simulink model "Modulador_torque"  (R2020b)
settings: Solver=ode23s  StartTime=0.0  StopTime=30  RelTol=1e-3
undefined symbols (not defined in the file): alfa_cu, Beq, Cts, Jeq, K_i_o, K_omega_o, K_tita_o, Kd, Ki, Kp, lambda_m, Ld, Lls, Lq, Pp, r, R0, R_Ref, Rd, Rq, Rts_amb, sigbuilder_block, TREF
libraries: simulink x2
settings Model: Creator=agustin  LastModifiedBy=emaag

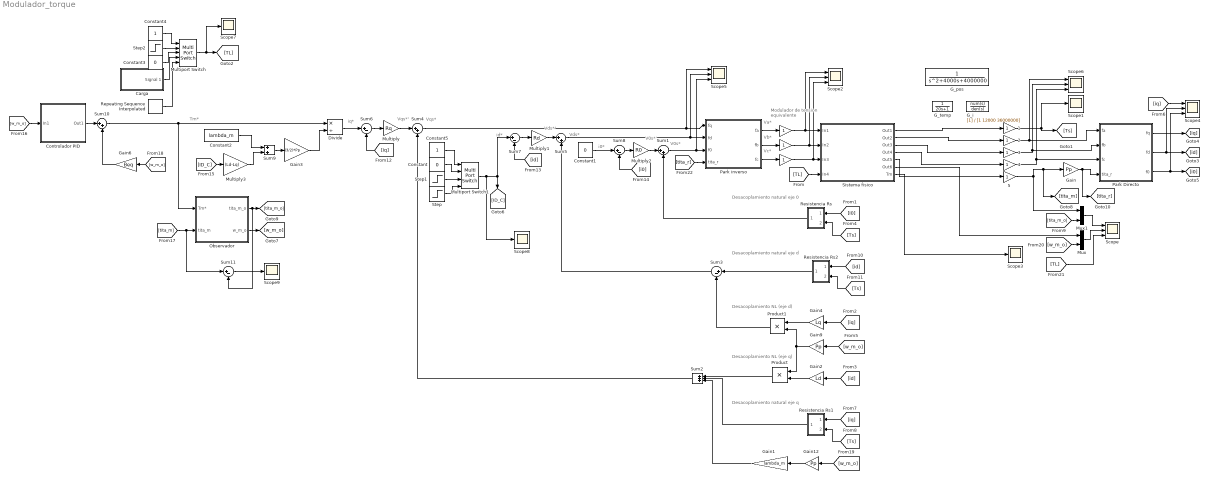
== system Modulador_torque ==
  note: Tm*
  note: V0s*'
  note: Vds*'
  note: Vqs*'
  note: i0*
  note: id*
  note: iq*
  note: V0s*
  note: Vds*
  note: Vb*
  note: Vc*
  note: Va*
  note: Desacoplamiento NL (eje q)
  note: Desacoplamiento NL (eje d)
  note: Vqs*
  note: Modulador de tension
      | equivalente
  note: Desacoplamiento natural eje 0
  note: Desacoplamiento natural eje q
  note: Desacoplamiento natural eje d
   {,,,1..5} (8 alike) : Gain
  Carga : Subsystem  Tag=STV Subsys  LoadFcn=sigbuilder_block('load');  StartFcn=sigbuilder_block('start');  StopFcn=sigbuilder_block('stop');  ClipboardFcn=sigbuilder_block('clipboard');  mask(Sigbuilder block){tuvar=[0:10]}
      mask help: Simulink:masks:SigbuilderBlock_MD
      mask init:
      | if ~strcmp(get_param(bdroot(gcbh),'SimulationStatus'),'stopped') tuvar = sigbuilder_block('maskInit'); end
      settings: CopyFcn=sigbuilder_block('copy');  DeleteFcn=sigbuilder_block('delete');  ModelCloseFcn=sigbuilder_block('modelClose');  PreSaveFcn=sigbuilder_block('preSave');  PauseFcn=sigbuilder_block('pause');  ContinueFcn=sigbuilder_block('continue');  NameChangeFcn=sigbuilder_block('namechange');  OpenFcn=sigbuilder_block('open',[6 30 1012.5 447.75 ]);  CloseFcn=sigbuilder_block('close');
      mask Display: plot(0, 0, 100, 100,[2, 2, 32, 32, 2], [68, 8, 8, 68, 68],[32, 2], [38, 38], [32, 19, 2],[53, 60, 44], [32, 17, 17, 2],[16, 16, 31, 31]);txt = getActiveGroup(gcbh);text(2, 100, txt,'verticalAlignment', 'top');
  Constant : Constant  Value=0
  Constant1 : Constant  Value=0
  Constant2 : Constant  Value=lambda_m
  Constant3 : Constant  Value=0
  Constant4 : Constant
  Constant5 : Constant
  Controlador PID : Subsystem
  Divide : Product  Inputs=*/
  G_i : TransferFcn  Denominator=[1 12000 36000000]
  G_pos : TransferFcn  Denominator=[1 4000 4000000]
  G_temp : TransferFcn  Denominator=[20 1]
  Gain : Gain  Gain=Pp
  Gain1 : Gain  Gain=lambda_m
  Gain12 : Gain  Gain=Pp
  Gain2 : Gain  Gain=Ld
  Gain3 : Gain  Gain=(3/2)*Pp
  Gain4 : Gain  Gain=Lq
  Gain6 : Gain  Gain=Beq
  Gain9 : Gain  Gain=Pp
  Multiply : Gain  Gain=Rq
  Multiply1 : Gain  Gain=Rd
  Multiply2 : Gain  Gain=R0
  Multiply3 : Gain  Gain=(Ld-Lq)
  Multiport Switch : MultiPortSwitch  Inputs=4
  Multiport Switch1 : MultiPortSwitch
  Mux : Mux  Inputs=2
  Mux1 : Mux  Inputs=2
  Observador : Subsystem
  Park Directo : MATLAB Function  TreatAsAtomicUnit=on
  Park inverso : MATLAB Function  TreatAsAtomicUnit=on
  Product : Product
  Product1 : Product
  Repeating Sequence Interpolated : simulink/Sources/Repeating Sequence Interpolated  OutValues="[0 0 6.28 6.28 -6.28 -6.28 0  0].'"  TimeValues="[0 .3 .30000001 .5 .5000001 .9 .9000001  10].'"  LookUpMeth=Interpolation-Use End Values  tsamp=0.01  OutMin=[]  OutMax=[]  OutDataTypeStr=double  OutputDataTypeScalingMode=double  OutDataType=fixdt(0,8)  OutScaling=2^-10
  Resistencia Rs : Subsystem
  Resistencia Rs1 : Subsystem
  Resistencia Rs2 : Subsystem
  Scope{,2,4..6} (5 alike) : Scope  NumInputPorts=3
  Scope{1,3,7..9} (5 alike) : Scope
  Sistema fisico : Subsystem
  Step : Step  Time=0.5  After=-1.9596  SampleTime=0
  Step1 : Step  Time=0.5  After=1.9596  SampleTime=0
  Step2 : Step  Time=3  After=6.28  SampleTime=0
  Sum{1,4..5,10} (4 alike) : Sum  Inputs=|++
  Sum{3,6..8,11} (5 alike) : Sum  Inputs=|+-
  Sum2 : Sum  Inputs=+++
  Sum9 : Sum
  wires:
  Sum5/1 -> Park inverso/2(fd), Scope5/2
  " 1"/1 -> [Ts], Scope1/1
  Gain4/1 -> Product1/1
  Park inverso/3(fc) -> " "/1
  Park inverso/1(fa) -> " "/1
  Sistema fisico/1(Out1) -> " 1"/1
  Park Directo/3(f0) -> Scope4/3, [i0]
  Sum1/1 -> Park inverso/3(f0), Scope5/3
  Gain/1 -> [tita_r], Park Directo/4(tita_r)
  [iq] -> Scope4/1
  Sistema fisico/4(Out4) -> " 4"/1
  [id] -> Gain2/1
  Sistema fisico/6(Out6) -> Mux/1
  " "/1 -> Scope2/2, Sistema fisico/2(In2)
  Sum4/1 -> Scope5/1, Park inverso/1(fq)
  [iq] -> Gain4/1
  " 3"/1 -> Scope6/2, Park Directo/2(fb)
  " "/1 -> Scope2/3, Sistema fisico/3(In3)
  [TL] -> Sistema fisico/4(In4)
  Sistema fisico/3(Out3) -> " 3"/1
  Park inverso/2(fb) -> " "/1
  " "/1 -> Sistema fisico/1(In1), Scope2/1
  Park Directo/2(fd) -> Scope4/2, [id]
  Sistema fisico/5(Out5) -> " 5"/1
  Sistema fisico/7(Tm) -> Scope3/1
  Gain2/1 -> Product/2
  " 4"/1 -> Scope6/3, Park Directo/3(fc)
  Sistema fisico/2(Out2) -> " 2"/1
  Park Directo/1(fq) -> [iq]
  " 2"/1 -> Scope6/1, Park Directo/1(fa)
  [i0] -> Resistencia Rs/1(In1)
  Resistencia Rs/1(In*Rs) -> Sum1/2
  [Ts] -> Resistencia Rs/2(Ts)
  [iq] -> Resistencia Rs1/1(In1)
  Resistencia Rs1/1(In*Rs) -> Sum2/2
  [Ts] -> Resistencia Rs1/2(Ts)
  Gain12/1 -> Gain1/1
  Sum2/1 -> Sum4/2
  [Ts] -> Resistencia Rs2/2(Ts)
  [id] -> Resistencia Rs2/1(In1)
  Sum3/1 -> Sum5/2
  Resistencia Rs2/1(In*Rs) -> Sum3/1
  Sum6/1 -> Multiply/1
  [iq] -> Sum6/2
  [id] -> Sum7/2
  [i0] -> Sum8/2
  Multiply/1 -> Sum4/1
  Multiply1/1 -> Sum5/1
  Sum7/1 -> Multiply1/1
  Sum8/1 -> Multiply2/1
  Multiply2/1 -> Sum1/1
  Product1/1 -> Sum3/2
  Product/1 -> Sum2/1
  Gain1/1 -> Sum2/3
  Step1/1 -> Multiport Switch1/3
  Constant/1 -> Multiport Switch1/2
  Step/1 -> Multiport Switch1/4
  Multiport Switch1/1 -> Scope8/1, [ID_C], Sum7/1
  Constant1/1 -> Sum8/1
  [ID_C] -> Multiply3/1
  Multiply3/1 -> Sum9/2
  Constant2/1 -> Sum9/1
  Sum9/1 -> Gain3/1
  Gain3/1 -> Divide/2
  Divide/1 -> Sum6/1
  Gain6/1 -> Sum10/2
  Constant3/1 -> Multiport Switch/3
  Carga/1(Signal 1) -> Multiport Switch/4
  Multiport Switch/1 -> Scope7/1, [TL]
  [w_m_o] -> Controlador PID/1(In1)
  " 5"/1 -> [tita_m], Gain/1, Mux1/1
  Sum10/1 -> Divide/1, Observador/1(Tm*)
  [w_m_o] -> Gain6/1
  [w_m_o] -> Gain9/1
  Gain9/1 -> Product1/2, Product/1
  [w_m_o] -> Gain12/1
  [tita_m_o] -> Mux1/2
  [w_m_o] -> Mux/2
  Mux1/1 -> Scope/1
  Mux/1 -> Scope/2
  [TL] -> Scope/3
  Step2/1 -> Multiport Switch/2
  Controlador PID/1(Out1) -> Sum10/1
  Constant4/1 -> Multiport Switch/1
  Constant5/1 -> Multiport Switch1/1
  [tita_m] -> Sum11/1, Observador/2(tita_m)
  Observador/1(tita_m_o) -> Sum11/2, [tita_m_o]
  Observador/2(w_m_o) -> [w_m_o]
  [tita_r] -> Park inverso/4(tita_r)
  Repeating Sequence Interpolated/1 -> Multiport Switch/5
  Sum11/1 -> Scope9/1

== system Modulador_torque/Carga ==
  Demux : Demux  Tag=STV Demux  Outputs=1
      settings: DisplayOption=none
  FromWs : FromWorkspace  Tag=STV FromWs  VariableName=tuvar
      SigBuilderData=|
      | common.afterFinalStr = 'Extrapolate'
      | common.sampleTime = 0
      | dataSet.timeRange = [0 10]
      | dataSet.name = 'Group 1'
      | sbobj.Groups.Name = 'Group 1'
      | sbobj.Groups.Signals.Name = 'Signal 1'
      | sbobj.Groups.Signals.XData = [0 0.3 0.3 0.5 0.5 0.9 0.9 10]
      | sbobj.Groups.Signals.YData = [0 0 6.28 6.28 -6.28 -6.28 0 0]
  Signal 1 : Outport  Tag=STV Outport  VectorParamsAs1DForOutWhenUnconnected=off
  wires:
  Demux/1 -> Signal 1/1
  FromWs/1 -> Demux/1

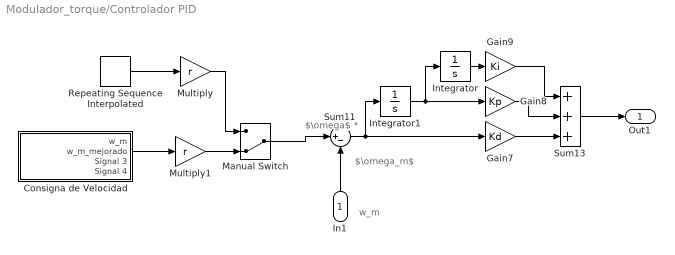
== system Modulador_torque/Controlador PID ==
  note: w_m
  note: $\omega_m$
  note: $\omega$ *
  In1 : Inport
  Consigna de Velocidad : Subsystem  Tag=STV Subsys  LoadFcn=sigbuilder_block('load');  StartFcn=sigbuilder_block('start');  StopFcn=sigbuilder_block('stop');  ClipboardFcn=sigbuilder_block('clipboard');  mask(Sigbuilder block){tuvar=[0:10]}
      mask help: Simulink:masks:SigbuilderBlock_MD
      mask init:
      | if ~strcmp(get_param(bdroot(gcbh),'SimulationStatus'),'stopped') tuvar = sigbuilder_block('maskInit'); end
      settings: CopyFcn=sigbuilder_block('copy');  DeleteFcn=sigbuilder_block('delete');  ModelCloseFcn=sigbuilder_block('modelClose');  PreSaveFcn=sigbuilder_block('preSave');  PauseFcn=sigbuilder_block('pause');  ContinueFcn=sigbuilder_block('continue');  NameChangeFcn=sigbuilder_block('namechange');  OpenFcn=sigbuilder_block('open',[6 30 1012.5 447.75 ]);  CloseFcn=sigbuilder_block('close');
      mask Display: plot(0, 0, 100, 100,[2, 2, 32, 32, 2], [68, 8, 8, 68, 68],[32, 2], [38, 38], [32, 19, 2],[53, 60, 44], [32, 17, 17, 2],[16, 16, 31, 31]);txt = getActiveGroup(gcbh);text(2, 100, txt,'verticalAlignment', 'top');
  Gain7 : Gain  Gain=Kd
  Gain8 : Gain  Gain=Kp
  Gain9 : Gain  Gain=Ki
  Integrator : Integrator
  Integrator1 : Integrator
  Manual Switch : ManualSwitch  CurrentSetting=0
  Multiply : Gain  Gain=r
  Multiply1 : Gain  Gain=r
  Repeating Sequence Interpolated : simulink/Sources/Repeating Sequence Interpolated  OutValues="[0 0 1.2566 1.2566 0  0 -1.2566 -1.2566 0 0].'"  TimeValues=[0 4.7 5 10 10.3 14.7 15 20 20.3 25].'  LookUpMeth=Interpolation-Use End Values  tsamp=0.01  OutMin=[]  OutMax=[]  OutDataTypeStr=double  OutputDataTypeScalingMode=double  OutDataType=fixdt(0,8)  OutScaling=2^-10
  Sum11 : Sum  Inputs=|+-
  Sum13 : Sum  Inputs=+++
  Out1 : Outport
  wires:
  Gain9/1 -> Sum13/1
  Sum11/1 -> Integrator1/1, Gain7/1
  Sum13/1 -> Out1/1
  Integrator1/1 -> Integrator/1, Gain8/1
  Gain8/1 -> Sum13/2
  Integrator/1 -> Gain9/1
  Gain7/1 -> Sum13/3
  In1/1 -> Sum11/2
  Manual Switch/1 -> Sum11/1
  Repeating Sequence Interpolated/1 -> Multiply/1
  Multiply/1 -> Manual Switch/1
  Consigna de Velocidad/2(w_m_mejorado) -> Multiply1/1
  Multiply1/1 -> Manual Switch/2

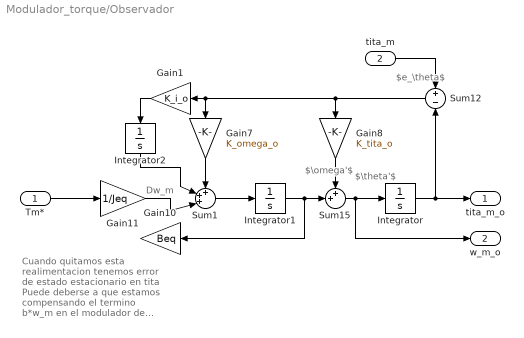
== system Modulador_torque/Observador ==
  note: $\omega'$
  note: $\theta'$
  note: $e_\theta$
  note: Cuando quitamos esta realimentacion tenemos error de estado estacionario en tita
      | Puede deberse a que estamos compensando el termino b*w_m en el modulador de torque
  note: Dw_m
  Tm* : Inport
  tita_m : Inport  Port=2
  Gain1 : Gain  Gain=K_i_o
  Gain10 : Gain  Gain=Beq
  Gain11 : Gain  Gain=1/Jeq
  Gain7 : Gain  Gain=K_omega_o
  Gain8 : Gain  Gain=K_tita_o
  Integrator : Integrator
  Integrator1 : Integrator
  Integrator2 : Integrator
  Sum1 : Sum  Inputs=+++|
  Sum12 : Sum  Inputs=+-
  Sum15 : Sum  Inputs=++|
  tita_m_o : Outport
  w_m_o : Outport  Port=2
  wires:
  Gain8/1 -> Sum15/1
  Integrator/1 -> tita_m_o/1, Sum12/2
  Sum1/1 -> Integrator1/1
  Integrator1/1 -> Sum15/2, Gain10/1
  Sum12/1 -> Gain1/1, Gain7/1, Gain8/1
  Sum15/1 -> w_m_o/1, Integrator/1
  tita_m/1 -> Sum12/1
  Tm*/1 -> Gain11/1
  Gain1/1 -> Integrator2/1
  Gain7/1 -> Sum1/1
  Integrator2/1 -> Sum1/2
  Gain11/1 -> Sum1/3

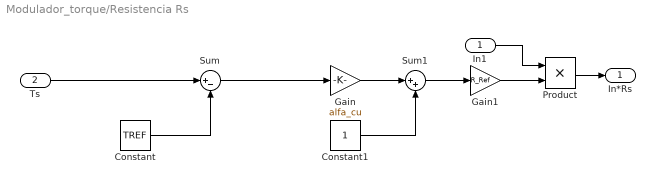
== system Modulador_torque/Resistencia Rs ==
  In1 : Inport
  Ts : Inport  Port=2
  Constant : Constant  Value=TREF
  Constant1 : Constant
  Gain : Gain  Gain=alfa_cu
  Gain1 : Gain  Gain=R_Ref
  Product : Product
  Sum : Sum  Inputs=|+-
  Sum1 : Sum  Inputs=|++
  In*Rs : Outport
  wires:
  Constant/1 -> Sum/2
  Gain/1 -> Sum1/1
  Gain1/1 -> Product/2
  Sum1/1 -> Gain1/1
  Sum/1 -> Gain/1
  Ts/1 -> Sum/1
  Constant1/1 -> Sum1/2
  In1/1 -> Product/1
  Product/1 -> In*Rs/1

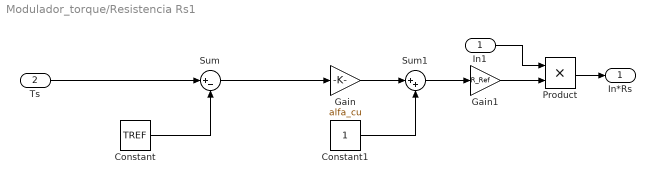
== system Modulador_torque/Resistencia Rs1 ==
  In1 : Inport
  Ts : Inport  Port=2
  Constant : Constant  Value=TREF
  Constant1 : Constant
  Gain : Gain  Gain=alfa_cu
  Gain1 : Gain  Gain=R_Ref
  Product : Product
  Sum : Sum  Inputs=|+-
  Sum1 : Sum  Inputs=|++
  In*Rs : Outport
  wires:
  Constant/1 -> Sum/2
  Gain/1 -> Sum1/1
  Gain1/1 -> Product/2
  Sum1/1 -> Gain1/1
  Sum/1 -> Gain/1
  Ts/1 -> Sum/1
  Constant1/1 -> Sum1/2
  In1/1 -> Product/1
  Product/1 -> In*Rs/1

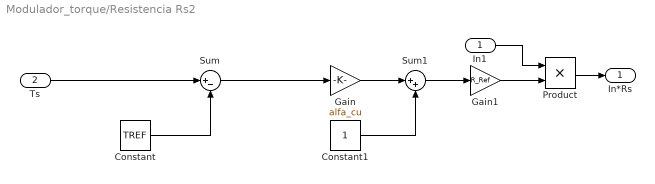
== system Modulador_torque/Resistencia Rs2 ==
  In1 : Inport
  Ts : Inport  Port=2
  Constant : Constant  Value=TREF
  Constant1 : Constant
  Gain : Gain  Gain=alfa_cu
  Gain1 : Gain  Gain=R_Ref
  Product : Product
  Sum : Sum  Inputs=|+-
  Sum1 : Sum  Inputs=|++
  In*Rs : Outport
  wires:
  Constant/1 -> Sum/2
  Gain/1 -> Sum1/1
  Gain1/1 -> Product/2
  Sum1/1 -> Gain1/1
  Sum/1 -> Gain/1
  Ts/1 -> Sum/1
  Constant1/1 -> Sum1/2
  In1/1 -> Product/1
  Product/1 -> In*Rs/1

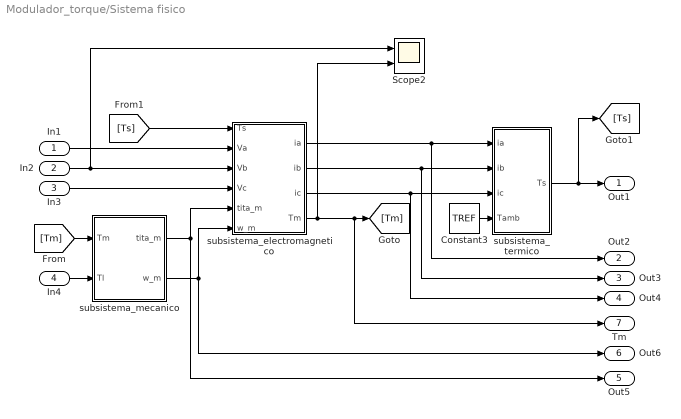
== system Modulador_torque/Sistema fisico ==
  In1 : Inport
  In2 : Inport  Port=2
  In3 : Inport  Port=3
  In4 : Inport  Port=4
  Constant3 : Constant  Value=TREF
  Scope2 : Scope  NumInputPorts=2
  "subsistema_electromagnetico " : Subsystem
  "subsistema_mecanico " : Subsystem
  subsistema_termico : Subsystem
  Out1 : Outport  VectorParamsAs1DForOutWhenUnconnected=off
  Out2 : Outport  Port=2  VectorParamsAs1DForOutWhenUnconnected=off
  Out3 : Outport  Port=3  VectorParamsAs1DForOutWhenUnconnected=off
  Out4 : Outport  Port=4  VectorParamsAs1DForOutWhenUnconnected=off
  Out5 : Outport  Port=5  VectorParamsAs1DForOutWhenUnconnected=off
  Out6 : Outport  Port=6  VectorParamsAs1DForOutWhenUnconnected=off
  Tm : Outport  Port=7  VectorParamsAs1DForOutWhenUnconnected=off
  wires:
  "subsistema_mecanico "/2(w_m) -> Out6/1, "subsistema_electromagnetico "/6(w_m)
  "subsistema_electromagnetico "/3(ic) -> Out4/1, subsistema_termico/3("ic ")
  In2/1 -> Scope2/1, "subsistema_electromagnetico "/3(Vb)
  [Tm] -> "subsistema_mecanico "/1(Tm)
  In4/1 -> "subsistema_mecanico "/2(Tl)
  "subsistema_electromagnetico "/1(ia) -> Out2/1, subsistema_termico/1(ia)
  "subsistema_electromagnetico "/4(Tm) -> Scope2/2, Tm/1, [Tm]
  In1/1 -> "subsistema_electromagnetico "/2(Va)
  Constant3/1 -> subsistema_termico/4(Tamb)
  "subsistema_electromagnetico "/2(ib) -> Out3/1, subsistema_termico/2(ib)
  In3/1 -> "subsistema_electromagnetico "/4(Vc)
  "subsistema_mecanico "/1("tita_m ") -> Out5/1, "subsistema_electromagnetico "/5(tita_m)
  subsistema_termico/1(Ts) -> [Ts], Out1/1
  [Ts] -> "subsistema_electromagnetico "/1(Ts)

== system Modulador_torque/Controlador PID/Consigna de Velocidad ==
  Demux : Demux  Tag=STV Demux
      settings: DisplayOption=none
  FromWs : FromWorkspace  Tag=STV FromWs  VariableName=tuvar
      SigBuilderData=|
      | common.afterFinalStr = 'Extrapolate'
      | common.sampleTime = 0
      | dataSet.timeRange = [0 25]
      | dataSet.name = 'Group 1'
      | sbobj.Groups.Name = 'Group 1'
      | sbobj.Groups.Signals(1).Name = 'w_m'
      | sbobj.Groups.Signals(1).XData = [0 5 5 10 10 15 15 20 20 25]
      | sbobj.Groups.Signals(1).YData = [0 0 1.2566 1.25660004683 0 0 -1.2566 -1.2566 0 0]
      | sbobj.Groups.Signals(2).Name = 'w_m_mejorado'
      | sbobj.Groups.Signals(2).XData = [0 4.7 5 10 10.3 14.7 15 20 20.3 25]
      | sbobj.Groups.Signals(2).YData = [0 0 1.25660004683 1.25660004683 0 0 -1.25660004683 -1.25660004683 0 0]
      | sbobj.Groups.Signals(3).Name = 'Signal 3'
      | sbobj.Groups.Signals(3).XData = [0 3.28 6 6 9 9 11.94 25]
      | sbobj.Groups.Signals(3).YData = [0 0 0 1 1 0 0 0]
      | sbobj.Groups.Signals(4).Name = 'Signal 4'
      | sbobj.Groups.Signals(4).XData = [0 6.8 6.8 10.2 10.2 25]
      | sbobj.Groups.Signals(4).YData = [0 0 1 1 0 0]
      | sbobj.Groups.TimeRange = [0 25]
  w_m : Outport  Tag=STV Outport  VectorParamsAs1DForOutWhenUnconnected=off
  w_m_mejorado : Outport  Tag=STV Outport  Port=2
  Signal 3 : Outport  Tag=STV Outport  Port=3
  Signal 4 : Outport  Tag=STV Outport  Port=4
  wires:
  Demux/1 -> w_m/1
  FromWs/1 -> Demux/1
  Demux/2 -> w_m_mejorado/1
  Demux/3 -> Signal 3/1
  Demux/4 -> Signal 4/1

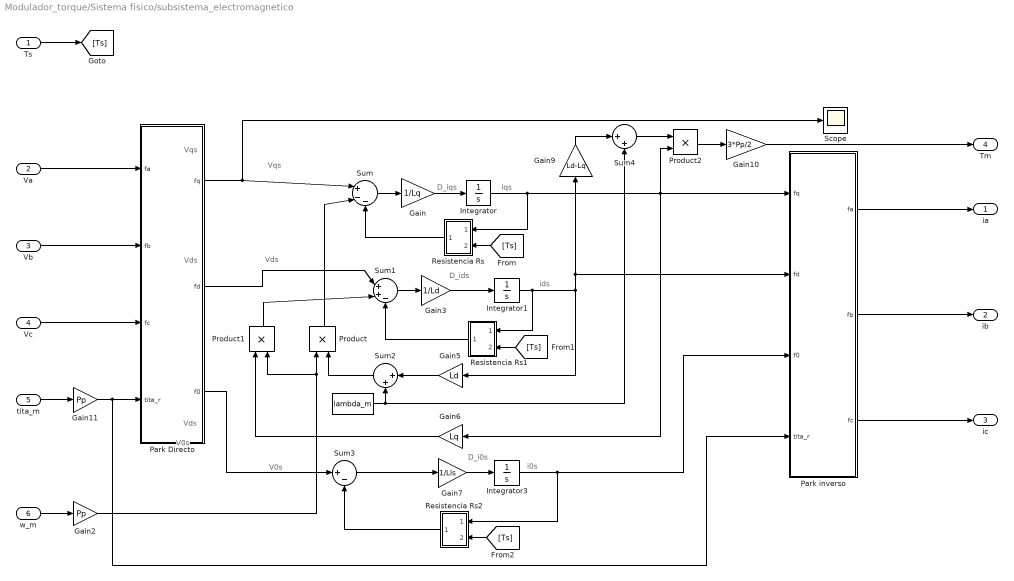
== system Modulador_torque/Sistema fisico/subsistema_electromagnetico  ==
  note: V0s
  note: Vds
  note: Vqs
  note: Vds
  note: Vqs
  note: V0s
  note: Vds
  note: i0s
  note: D_i0s
  note: D_ids
  note: ids
  note: iqs
  note: D_iqs
  Ts : Inport
  Va : Inport  Port=2
  Vb : Inport  Port=3
  Vc : Inport  Port=4
  tita_m : Inport  Port=5
  w_m : Inport  Port=6
  " " : Constant  Value=lambda_m
  Gain : Gain  Gain=1/Lq
  Gain10 : Gain  Gain=3*Pp/2
  Gain11 : Gain  Gain=Pp
  Gain2 : Gain  Gain=Pp
  Gain3 : Gain  Gain=1/Ld
  Gain5 : Gain  Gain=Ld
  Gain6 : Gain  Gain=Lq
  Gain7 : Gain  Gain=1/Lls
  Gain9 : Gain  Gain=Ld-Lq
  Integrator : Integrator
  Integrator1 : Integrator
  Integrator3 : Integrator
  Park Directo : MATLAB Function  TreatAsAtomicUnit=on
  Park inverso : MATLAB Function  TreatAsAtomicUnit=on
  Product : Product
  Product1 : Product
  Product2 : Product
  Resistencia Rs : Subsystem
  Resistencia Rs1 : Subsystem
  Resistencia Rs2 : Subsystem
  Scope : Scope
  Sum : Sum  Inputs=|+--
  Sum1 : Sum  Inputs=|++-
  Sum2 : Sum  Inputs=|++
  Sum3 : Sum  Inputs=|+-
  Sum4 : Sum  Inputs=|++
  ia : Outport  VectorParamsAs1DForOutWhenUnconnected=off
  ib : Outport  Port=2  VectorParamsAs1DForOutWhenUnconnected=off
  ic : Outport  Port=3  VectorParamsAs1DForOutWhenUnconnected=off
  Tm : Outport  Port=4  VectorParamsAs1DForOutWhenUnconnected=off
  wires:
  Product/1 -> Sum/2
  w_m/1 -> Gain2/1
  Product1/1 -> Sum1/2
  Gain2/1 -> Product1/2, Product/1
  Park Directo/3(f0) -> Sum3/1
  Integrator/1 -> Resistencia Rs/1(In1), Product2/2, Park inverso/1(fq), Gain6/1
  Sum2/1 -> Product/2
  Sum3/1 -> Gain7/1
  Park Directo/1(fq) -> Scope/1, Sum/1
  Sum/1 -> Gain/1
  Gain3/1 -> Integrator1/1
  Park Directo/2(fd) -> Sum1/1
  Sum1/1 -> Gain3/1
  Gain5/1 -> Sum2/1
  Gain/1 -> Integrator/1
  Gain6/1 -> Product1/1
  Resistencia Rs/1(In*Rs) -> Sum/3
  " "/1 -> Sum4/2, Sum2/2
  Gain7/1 -> Integrator3/1
  Gain9/1 -> Sum4/1
  Sum4/1 -> Product2/1
  Product2/1 -> Gain10/1
  Gain10/1 -> Tm/1
  Vb/1 -> Park Directo/2(fb)
  Va/1 -> Park Directo/1(fa)
  Vc/1 -> Park Directo/3(fc)
  tita_m/1 -> Gain11/1
  Gain11/1 -> Park inverso/4(tita_r), Park Directo/4(tita_r)
  Park inverso/1(fa) -> ia/1
  Park inverso/2(fb) -> ib/1
  Park inverso/3(fc) -> ic/1
  Ts/1 -> [Ts]
  [Ts] -> Resistencia Rs/2(Ts)
  Resistencia Rs1/1(In*Rs) -> Sum1/3
  Integrator1/1 -> Gain9/1, Park inverso/2(fd), Gain5/1, Resistencia Rs1/1(In1)
  [Ts] -> Resistencia Rs1/2(Ts)
  Resistencia Rs2/1(In*Rs) -> Sum3/2
  Integrator3/1 -> Resistencia Rs2/1(In1), Park inverso/3(f0)
  [Ts] -> Resistencia Rs2/2(Ts)

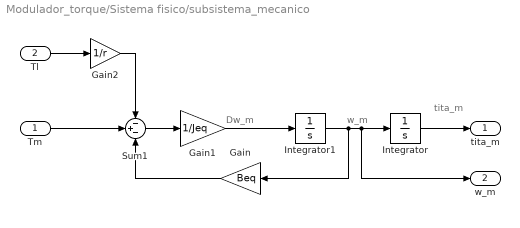
== system Modulador_torque/Sistema fisico/subsistema_mecanico  ==
  note: Dw_m
  note: w_m
  note: tita_m
  Tm : Inport
  Tl : Inport  Port=2
  Gain : Gain  Gain=Beq
  Gain1 : Gain  Gain=1/Jeq
  Gain2 : Gain  Gain=1/r
  Integrator : Integrator
  Integrator1 : Integrator
  Sum1 : Sum  Inputs=-+-
  "tita_m " : Outport  VectorParamsAs1DForOutWhenUnconnected=off
  w_m : Outport  Port=2  VectorParamsAs1DForOutWhenUnconnected=off
  wires:
  Gain1/1 -> Integrator1/1
  Integrator1/1 -> Integrator/1, w_m/1, Gain/1
  Integrator/1 -> "tita_m "/1
  Sum1/1 -> Gain1/1
  Gain/1 -> Sum1/3
  Tm/1 -> Sum1/2
  Tl/1 -> Gain2/1
  Gain2/1 -> Sum1/1

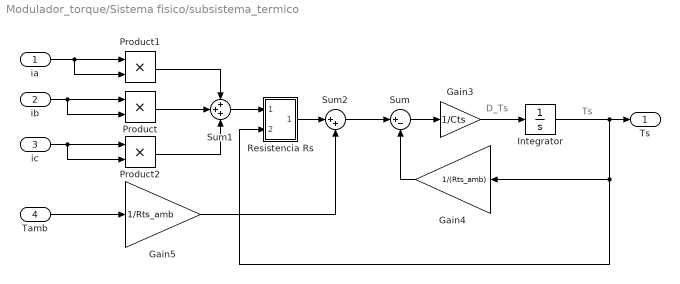
== system Modulador_torque/Sistema fisico/subsistema_termico ==
  note: Ts
  note: D_Ts
  ia : Inport
  ib : Inport  Port=2
  "ic " : Inport  Port=3
  Tamb : Inport  Port=4
  Gain3 : Gain  Gain=1/Cts
  Gain4 : Gain  Gain=1/(Rts_amb)
  Gain5 : Gain  Gain=1/Rts_amb
  Integrator : Integrator  InitialCondition=40
  Product : Product
  Product1 : Product
  Product2 : Product
  Resistencia Rs : Subsystem
  Sum : Sum  Inputs=|+-
  Sum1 : Sum  Inputs=+++
  Sum2 : Sum  Inputs=|++
  Ts : Outport  VectorParamsAs1DForOutWhenUnconnected=off
  wires:
  Gain4/1 -> Sum/2
  Sum1/1 -> Resistencia Rs/1(In1)
  Product2/1 -> Sum1/3
  Product/1 -> Sum1/2
  Integrator/1 -> Ts/1, Resistencia Rs/2(Ts), Gain4/1
  ib/1 -> Product/2, Product/1
  "ic "/1 -> Product2/2, Product2/1
  Sum2/1 -> Sum/1
  Product1/1 -> Sum1/1
  Gain5/1 -> Sum2/2
  Resistencia Rs/1(In*Rs) -> Sum2/1
  ia/1 -> Product1/2, Product1/1
  Tamb/1 -> Gain5/1
  Gain3/1 -> Integrator/1
  Sum/1 -> Gain3/1

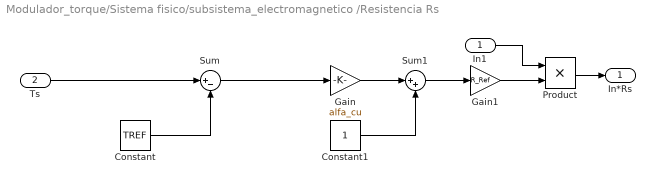
== system Modulador_torque/Sistema fisico/subsistema_electromagnetico /Resistencia Rs ==
  In1 : Inport
  Ts : Inport  Port=2
  Constant : Constant  Value=TREF
  Constant1 : Constant
  Gain : Gain  Gain=alfa_cu
  Gain1 : Gain  Gain=R_Ref
  Product : Product
  Sum : Sum  Inputs=|+-
  Sum1 : Sum  Inputs=|++
  In*Rs : Outport
  wires:
  Constant/1 -> Sum/2
  Gain/1 -> Sum1/1
  Gain1/1 -> Product/2
  Sum1/1 -> Gain1/1
  Sum/1 -> Gain/1
  Ts/1 -> Sum/1
  Constant1/1 -> Sum1/2
  In1/1 -> Product/1
  Product/1 -> In*Rs/1

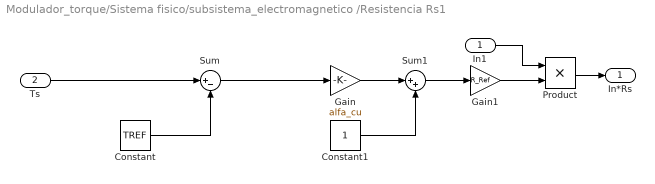
== system Modulador_torque/Sistema fisico/subsistema_electromagnetico /Resistencia Rs1 ==
  In1 : Inport
  Ts : Inport  Port=2
  Constant : Constant  Value=TREF
  Constant1 : Constant
  Gain : Gain  Gain=alfa_cu
  Gain1 : Gain  Gain=R_Ref
  Product : Product
  Sum : Sum  Inputs=|+-
  Sum1 : Sum  Inputs=|++
  In*Rs : Outport
  wires:
  Constant/1 -> Sum/2
  Gain/1 -> Sum1/1
  Gain1/1 -> Product/2
  Sum1/1 -> Gain1/1
  Sum/1 -> Gain/1
  Ts/1 -> Sum/1
  Constant1/1 -> Sum1/2
  In1/1 -> Product/1
  Product/1 -> In*Rs/1

== system Modulador_torque/Sistema fisico/subsistema_electromagnetico /Resistencia Rs2 ==
  In1 : Inport
  Ts : Inport  Port=2
  Constant : Constant  Value=TREF
  Constant1 : Constant
  Gain : Gain  Gain=alfa_cu
  Gain1 : Gain  Gain=R_Ref
  Product : Product
  Sum : Sum  Inputs=|+-
  Sum1 : Sum  Inputs=|++
  In*Rs : Outport
  wires:
  Constant/1 -> Sum/2
  Gain/1 -> Sum1/1
  Gain1/1 -> Product/2
  Sum1/1 -> Gain1/1
  Sum/1 -> Gain/1
  Ts/1 -> Sum/1
  Constant1/1 -> Sum1/2
  In1/1 -> Product/1
  Product/1 -> In*Rs/1

== system Modulador_torque/Sistema fisico/subsistema_termico/Resistencia Rs ==
  In1 : Inport
  Ts : Inport  Port=2
  Constant : Constant  Value=TREF
  Constant1 : Constant
  Gain : Gain  Gain=alfa_cu
  Gain1 : Gain  Gain=R_Ref
  Product : Product
  Sum : Sum  Inputs=|+-
  Sum1 : Sum  Inputs=|++
  In*Rs : Outport
  wires:
  Constant/1 -> Sum/2
  Gain/1 -> Sum1/1
  Gain1/1 -> Product/2
  Sum1/1 -> Gain1/1
  Sum/1 -> Gain/1
  Ts/1 -> Sum/1
  Constant1/1 -> Sum1/2
  In1/1 -> Product/1
  Product/1 -> In*Rs/1

== matlab function Modulador_torque/Park inverso ==
  data: fq input; fd input; f0 input; tita_r input; fa output; fb output; fc output
function [fa, fb, fc] = t_park_inv(fq, fd , f0, tita_r)


park_MATRIZ = [cos(tita_r)        sin(tita_r)        1; 
               cos(tita_r-2*pi/3) sin(tita_r-2*pi/3) 1;
               cos(tita_r+2*pi/3) sin(tita_r+2*pi/3) 1];
                 
park_inv = park_MATRIZ * [fq;fd;f0];
fa = park_inv(1);
fb = park_inv(2);
fc = park_inv(3);
end

== matlab function Modulador_torque/Sistema fisico/subsistema_electromagnetico /Park Directo ==
  data: fa input; fq output; fb input; fc input; tita_r input; fd output; f0 output
function [fq,fd,f0]     = t_park(fa,fb,fc,tita_r)

park_MATRIZ = [cos(tita_r) cos(tita_r-2*pi/3) cos(tita_r+2*pi/3); 
               sin(tita_r) sin(tita_r-2*pi/3) sin(tita_r+2*pi/3);
                  0.5           0.5            0.5];
                 
park_dir = (2/3) * park_MATRIZ * [fa;fb;fc];
fq = park_dir(1);
fd = park_dir(2);
f0 = park_dir(3);

end

== matlab function Modulador_torque/Sistema fisico/subsistema_electromagnetico /Park inverso ==
  data: fq input; fd input; f0 input; tita_r input; fa output; fb output; fc output
function [fa, fb, fc] = t_park_inv(fq, fd , f0, tita_r)


park_MATRIZ = [cos(tita_r)        sin(tita_r)        1; 
               cos(tita_r-2*pi/3) sin(tita_r-2*pi/3) 1;
               cos(tita_r+2*pi/3) sin(tita_r+2*pi/3) 1];
                 
park_inv = park_MATRIZ * [fq;fd;f0];
fa = park_inv(1);
fb = park_inv(2);
fc = park_inv(3);
end

== matlab function Modulador_torque/Park Directo ==
  data: fa input; fq output; fb input; fc input; tita_r input; fd output; f0 output
function [fq,fd,f0]     = t_park(fa,fb,fc,tita_r)

park_MATRIZ = [cos(tita_r) cos(tita_r-2*pi/3) cos(tita_r+2*pi/3); 
               sin(tita_r) sin(tita_r-2*pi/3) sin(tita_r+2*pi/3);
                  0.5           0.5            0.5];
                 
park_dir = (2/3) * park_MATRIZ * [fa;fb;fc];
fq = park_dir(1);
fd = park_dir(2);
f0 = park_dir(3);
end
